simulink model "modelo_NL_DH_GUIA"  (R2025b)
settings: Solver=ode4  StartTime=0.0  StopTime=TimeXP  FixedStep=0.005  RelTol=1e-3
values from neighbouring files (symbols this model uses):
  h_ref = he    [NL_missao.m]    (also in XP_inicializacao.m = h_now; XP_missao.m = XP_msl0; XP_voo.m = XP_msl0)
  h_ref0 = h_ref    [NL_missao.m]    (also in XP_doublets_lqry2.m = 600; XP_missao.m; XP_missao_lqry.m = XP_h_ref0; XP_missao_lqry2.m = XP_h_ref0)
  h_step_final = m.h_A    [G5_sil.m]    (also in XP_voo.m = cfg(7))
  h_step_t = m.h_t(1)    [G5_sil.m]    (also in XP_voo.m = cfg(8))
  h_step_t2 = m.h_t(2)    [G5_sil.m]    (also in XP_voo.m = cfg(13))
  h_step_t3 = m.h_t(3)    [G5_sil.m]    (also in XP_voo.m = cfg(14))
  he = h_now    [XP_inicializacao.m]    (also in XP_missao.m = XP_msl0; XP_voo.m = XP_msl0)
  Kp = 0.40    (= 0.4)    [VR_replay_xp.m]    (also in XPL_probe_lat.m)
  Kq = 0.50    (= 0.5)    [VR_replay_xp.m]    (also in XPL_probe_lat.m; XP_retune_Ctheta.m = 0.1)
  psi_ref_final = deg2rad(m.psi_A)    [G5_sil.m]    (also in XP_voo.m = deg2rad(cfg(9)))
  psi_ref_t = m.psi_t(1)    [G5_sil.m]    (also in XP_voo.m = cfg(10))
  psi_ref_t2 = m.psi_t(2)    [G5_sil.m]    (also in XP_voo.m = cfg(15))
  psi_ref_t3 = m.psi_t(3)    [G5_sil.m]    (also in XP_voo.m = cfg(16))
  R_accept = cfgm.R    [NL_missao.m]    (also in XP_doublets_lqry2.m = 80; XP_missao.m = XP_R_accept; XP_missao_lqry.m = cfg_user.R; XP_missao_lqry2.m = cfg_user.R)
  theta_ref_clamp = [-0.1745  deg2rad(3)]    [XP_missao.m]    (also in XP_voo.m)
  theta_test_final = 0    [NL_missao.m]    (also in XP_missao.m = cfgm.thf)
  theta_test_init = 0    [NL_missao.m]    (also in XP_missao.m)
  theta_test_t = 1e9    (= 1000000000)    [NL_missao.m]    (also in XP_missao.m = cfgm.tht)
  TrimInput = [ctrl(4);               ctrl(1)*max_deflection;               ctrl(2)*max_deflection;               ctrl(3)*max_deflection]    [XP_inicializacao.m]    (also in XP_missao.m = [0.43; deg2rad(7.0); 0; 0]; XP_voo.m = [0.43; Ue(2); 0; 0])
  VT_ref = Ve    [NL_missao.m]    (also in XP_inicializacao.m; XP_missao.m; XP_voo.m)
  VT_ref0 = VT_ref    [NL_missao.m]    (also in XP_doublets_lqry2.m = XP_dbl_VT; XP_missao.m; XP_missao_lqry.m = 12; XP_missao_lqry2.m = 12)
  VT_step_delta = m.VT_delta    [G5_sil.m]    (also in XP_voo.m = cfg(11))
  VT_step_t = m.VT_t    [G5_sil.m]    (also in XP_voo.m = cfg(12))
  WPs = WPs_user(1,:)    [NL_missao.m]    (also in XP_doublets_lqry2.m = WPs_user; WPs(:,1:2) = ne'; XP_missao.m; XP_missao_lqry.m; XP_missao_lqry2.m)
  Xe = montaX(y)    [VR_plot_sato_real.m]    (also in VR_tic.m; plot_degrau_3vias_sato.m)
undefined symbols (not defined in the file or in its folder): act, C_alt, C_phi, C_theta, C_vel, eng, h_step_init, K_heading, Kr, psi_ref_init, tau_ref, Ve
libraries: slpidlib x4, hdlsllib x1
settings Model: Creator=anade  LastModifiedBy=kaue
settings SolverCC: ZeroCrossAlgorithm=Adaptive
settings DebuggingCC: AlgebraicLoopMsg=none  IgnoredZcDiagnostic=none

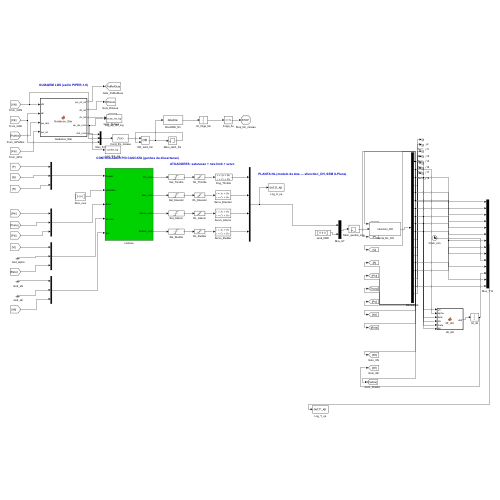
[thumbnail: Simulink's stored preview of the top-level diagram]
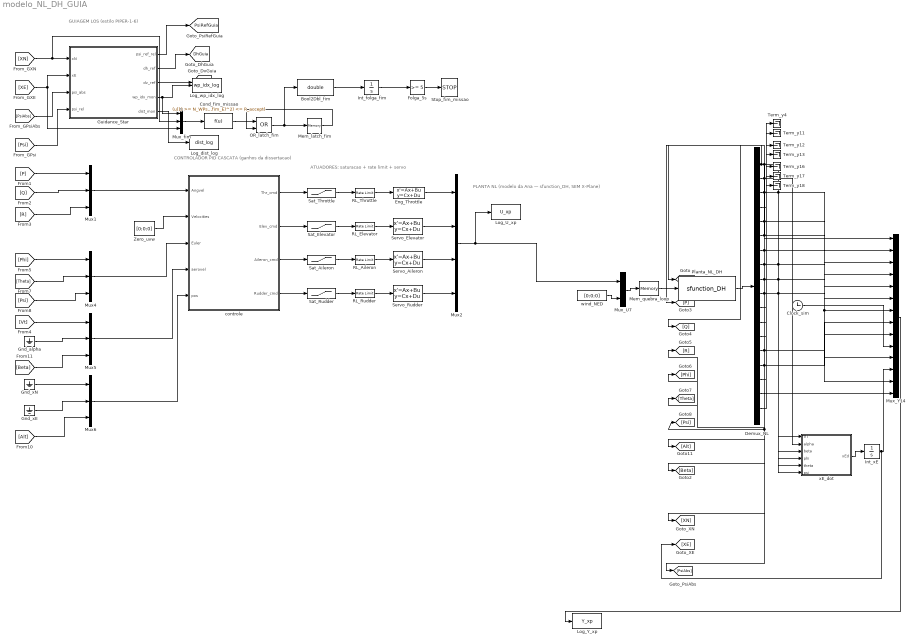
== system modelo_NL_DH_GUIA ==
  note: GUIAGEM LOS (estilo PIPER-1-6)
  note: CONTROLADOR PID CASCATA (ganhos da dissertacao)
  note: ATUADORES: saturacao + rate limit + servo
  note: PLANTA NL (modelo da Ana — sfunction_DH, SEM X-Plane)
  Bool2Dbl_fim : DataTypeConversion  OutDataTypeStr=double
  Clock_sim : Clock
  Cond_fim_missao : Fcn  Expr=(u(1) >= N_WPs) && (sqrt((u(2)-WPfim_N)^2 + (u(3)-WPfim_E)^2) <= R_accept)
  Demux_NL : Demux  Outputs=18
  Eng_Throttle : StateSpace  A=-1/eng.tau  B=1/eng.tau  D=0  InitialCondition=TrimInput(1)
  Folga_5s : hdlsllib/Logic and Bit Operations/Compare To Constant  relop=>=  const=5  OutDataTypeStr=boolean
  Gnd_alpha : Ground
  Gnd_xE : Ground
  Gnd_xN : Ground
  Guidance_Star : MATLAB Function  TreatAsAtomicUnit=on
  Int_folga_fim : Integrator
  Int_xE : Integrator
  Log_U_xp : ToWorkspace  VariableName=U_xp
  Log_Y_xp : ToWorkspace  VariableName=Y_xp
  Log_dist_log : ToWorkspace  VariableName=dist_log  SampleTime=-1
  Log_wp_idx_log : ToWorkspace  VariableName=wp_idx_log  SampleTime=-1
  Mem_latch_fim : Memory
  Mem_quebra_loop : Memory
  Mux{1,4..6} (4 alike) : Mux  Inputs=3
  Mux2 : Mux
  Mux_U7 : Mux  Inputs=2
  Mux_Y14 : Mux  Inputs=14
  Mux_fim : Mux  Inputs=3
  OR_latch_fim : Logic  Operator=OR  AllPortsSameDT=off  OutDataTypeStr=boolean
  Planta_NL_DH : S-Function  FunctionName=sfunction_DH  Parameters=Xe  SFunctionDeploymentMode=off  EnableBusSupport=off
  RL_Aileron : RateLimiter  RisingSlewLimit=act.rate  FallingSlewLimit=-act.rate  InitialCondition=TrimInput(3)
  RL_Elevator : RateLimiter  RisingSlewLimit=act.rate  FallingSlewLimit=-act.rate  InitialCondition=TrimInput(2)
  RL_Rudder : RateLimiter  RisingSlewLimit=act.rate  FallingSlewLimit=-act.rate  InitialCondition=TrimInput(4)
  RL_Throttle : RateLimiter  RisingSlewLimit=eng.rate  FallingSlewLimit=-eng.rate  InitialCondition=TrimInput(1)
  Sat_Aileron : Saturate  UpperLimit=0.4363  LowerLimit=-0.4363
  Sat_Elevator : Saturate  UpperLimit=0.4363  LowerLimit=-0.4363
  Sat_Rudder : Saturate  UpperLimit=0.4363  LowerLimit=-0.4363
  Sat_Throttle : Saturate  UpperLimit=1  LowerLimit=0
  Servo_Aileron : StateSpace  A=-act.bw  B=act.bw  D=0  InitialCondition=TrimInput(3)
  Servo_Elevator : StateSpace  A=-act.bw  B=act.bw  D=0  InitialCondition=TrimInput(2)
  Servo_Rudder : StateSpace  A=-act.bw  B=act.bw  D=0  InitialCondition=TrimInput(4)
  Stop_fim_missao : Stop
  Term_y{4,11..13,16..18} (7 alike) : Terminator
  Zero_uvw : Constant  Value=[0;0;0]
  controle : Subsystem
  wind_NED : Constant  Value=[0;0;0]
  xE_dot : MATLAB Function  TreatAsAtomicUnit=on
  tag scope: DhGuia=global, DvGuia=global, PsiRefGuia=global
  wires:
  [XN] -> Mux_fim/2, Guidance_Star/1(xN)
  [XE] -> Guidance_Star/2(xE), Mux_fim/3
  Sat_Throttle/1 -> RL_Throttle/1
  [P] -> Mux1/1
  [PsiAbs] -> Guidance_Star/3(psi_abs)
  [R] -> Mux1/3
  [Q] -> Mux1/2
  [Psi] -> Guidance_Star/4(psi_rel)
  [Phi] -> Mux4/1
  [Theta] -> Mux4/2
  [Psi] -> Mux4/3
  [Vt] -> Mux5/1
  Gnd_xN/1 -> Mux6/1
  Gnd_alpha/1 -> Mux5/2
  Mux4/1 -> controle/3(Euler)
  [Beta] -> Mux5/3
  controle/2(Elev_cmd) -> Sat_Elevator/1
  Mux5/1 -> controle/4(aerovel)
  Gnd_xE/1 -> Mux6/2
  Sat_Aileron/1 -> RL_Aileron/1
  [Alt] -> Mux6/3
  Guidance_Star/1(psi_ref_rel) -> [PsiRefGuia]
  Guidance_Star/2(dh_ref) -> [DhGuia]
  Sat_Rudder/1 -> RL_Rudder/1
  Mux1/1 -> controle/1(Angvel)
  Mux6/1 -> controle/5(pos)
  Zero_uvw/1 -> controle/2(Velocities)
  controle/1(Thr_cmd) -> Sat_Throttle/1
  controle/3(Aileron_cmd) -> Sat_Aileron/1
  controle/4(Rudder_cmd) -> Sat_Rudder/1
  Sat_Elevator/1 -> RL_Elevator/1
  Servo_Elevator/1 -> Mux2/2
  RL_Throttle/1 -> Eng_Throttle/1
  Eng_Throttle/1 -> Mux2/1
  RL_Elevator/1 -> Servo_Elevator/1
  RL_Aileron/1 -> Servo_Aileron/1
  RL_Rudder/1 -> Servo_Rudder/1
  Servo_Aileron/1 -> Mux2/3
  Servo_Rudder/1 -> Mux2/4
  Mux2/1 -> Log_U_xp/1, Mux_U7/1
  wind_NED/1 -> Mux_U7/2
  Mux_U7/1 -> Mem_quebra_loop/1
  Mem_quebra_loop/1 -> Planta_NL_DH/1
  Planta_NL_DH/1 -> Demux_NL/1
  Demux_NL/1 -> xE_dot/1(VT), Mux_Y14/1, [Vt]
  Demux_NL/3 -> xE_dot/3(beta), Mux_Y14/9, [Beta]
  Demux_NL/5 -> [P], Mux_Y14/2
  Demux_NL/6 -> [Q], Mux_Y14/3
  Demux_NL/7 -> [R], Mux_Y14/4
  Demux_NL/8 -> xE_dot/4(phi), Mux_Y14/5, [Phi]
  Demux_NL/9 -> xE_dot/5(theta), Mux_Y14/6, [Theta]
  Demux_NL/10 -> [Psi], [PsiAbs], Mux_Y14/7, Mux_Y14/13, xE_dot/6(psi)
  Demux_NL/14 -> [XN], Mux_Y14/11
  Demux_NL/15 -> [Alt], Mux_Y14/8
  Demux_NL/2 -> xE_dot/2(alpha), Mux_Y14/14
  xE_dot/1(xEd) -> Int_xE/1
  Int_xE/1 -> [XE], Mux_Y14/12
  Demux_NL/4 -> Term_y4/1
  Demux_NL/11 -> Term_y11/1
  Demux_NL/12 -> Term_y12/1
  Demux_NL/13 -> Term_y13/1
  Demux_NL/16 -> Term_y16/1
  Demux_NL/17 -> Term_y17/1
  Demux_NL/18 -> Term_y18/1
  Clock_sim/1 -> Mux_Y14/10
  Mux_Y14/1 -> Log_Y_xp/1
  Guidance_Star/3(dv_ref) -> [DvGuia]
  Guidance_Star/4(wp_idx_mon) -> Mux_fim/1, Log_wp_idx_log/1
  Guidance_Star/5(dist_mon) -> Log_dist_log/1
  Mux_fim/1 -> Cond_fim_missao/1
  Cond_fim_missao/1 -> OR_latch_fim/1
  Mem_latch_fim/1 -> OR_latch_fim/2
  OR_latch_fim/1 -> Bool2Dbl_fim/1, Mem_latch_fim/1
  Bool2Dbl_fim/1 -> Int_folga_fim/1
  Int_folga_fim/1 -> Folga_5s/1
  Folga_5s/1 -> Stop_fim_missao/1

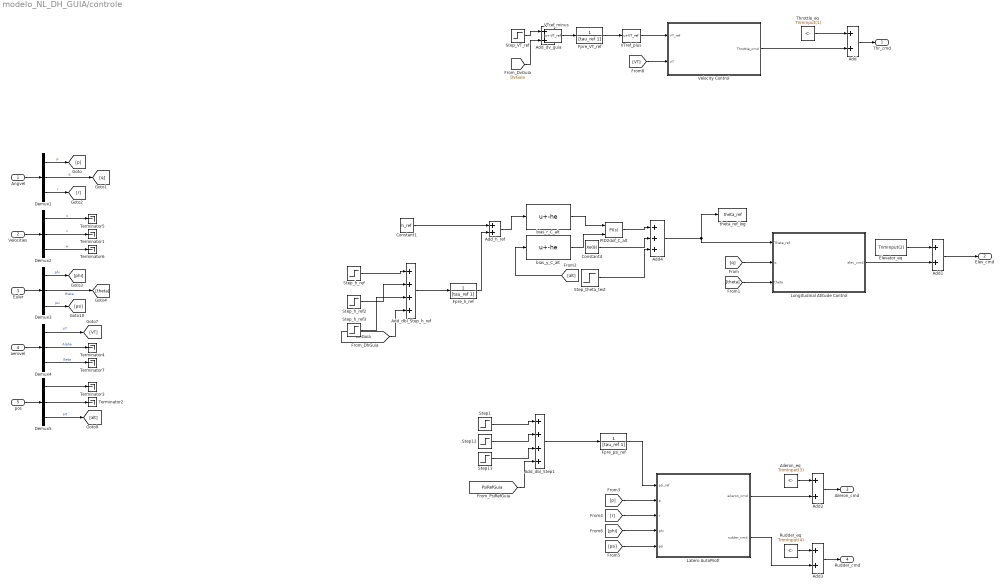
== system modelo_NL_DH_GUIA/controle ==
  Angvel : Inport
  Velocities : Inport  Port=2
  Euler : Inport  Port=3
  aerovel : Inport  Port=4
  pos : Inport  Port=5
  Add{,1..3} (4 alike) : Sum
  Add4 : Sum  Inputs=+++
  Add_dbl_Step1 : Sum  Inputs=++++
  Add_dbl_Step_h_ref : Sum  Inputs=++++
  Add_dv_guia : Sum
  Add_h_ref : Sum
  Aileron_eq : Constant  Value=TrimInput(3)
  Constant1 : Constant  Value=h_ref
  Constant4 : Constant  Value=Xe(8)
  Demux{1..5} (5 alike) : Demux  Outputs=3
  Elevator_eq : Constant  Value=TrimInput(2)
  Fpre_VT_ref : TransferFcn  Denominator=[tau_ref 1]
  Fpre_h_ref : TransferFcn  Denominator=[tau_ref 1]
  Fpre_psi_ref : TransferFcn  Denominator=[tau_ref 1]
  Latero AutoPilotl : Subsystem
  Longitudinal Atitude Control : Subsystem
  PID2dof_C_alt : slpidlib/PID Controller (2DOF)  Controller=PI  Form=Parallel  TimeDomain=Continuous-time  UseExternalTs=off  SampleTime=-1  IntegratorMethod=Forward Euler  FilterMethod=Forward Euler  ControllerParametersSource=internal  P=C_alt.Kp  I=C_alt.Ki  UseKiTs=off  D=0  UseExternalDerivativeSource=off  N=100  UseFilter=on  b=0  c=1  TunerSelectOption=Transfer Function Based (PID Tuner App)  InitialConditionSource=internal  InitialConditionForIntegrator=0  InitialConditionForFilter=0  DifferentiatorICPrevScaledInput=0  ExternalReset=none  TrackingMode=off  Kt=1  LimitOutput=on  SatLimitsSource=internal  UpperSaturationLimit=theta_ref_clamp(2)  LowerSaturationLimit=theta_ref_clamp(1)  LinearizeAsGain=on  AntiWindupMode=clamping  Kb=1  LimitIntegrator=off  UpperIntegratorSaturationLimit=inf  LowerIntegratorSaturationLimit=-inf  POutMin=[]  POutMax=[]  IOutMin=[]  IOutMax=[]  DOutMin=[]  DOutMax=[]  NOutMin=[]  NOutMax=[]  bOutMin=[]  bOutMax=[]  cOutMin=[]  cOutMax=[]  SumOutMin=[]  SumOutMax=[]  SaturationOutMin=[]  SaturationOutMax=[]  PParamMin=[]  PParamMax=[]  IParamMin=[]  IParamMax=[]  DParamMin=[]  DParamMax=[]  NParamMin=[]  NParamMax=[]  bParamMin=[]  bParamMax=[]  cParamMin=[]  cParamMax=[]  KbParamMin=[]  KbParamMax=[]  KtParamMin=[]  KtParamMax=[]  KbOutMin=[]  KbOutMax=[]  KtOutMin=[]  KtOutMax=[]  IntegratorOutMin=[]  IntegratorOutMax=[]  FilterOutMin=[]  FilterOutMax=[]  SumI1OutMin=[]  SumI1OutMax=[]  SumI2OutMin=[]  SumI2OutMax=[]  SumI3OutMin=[]  SumI3OutMax=[]  SumI4OutMin=[]  SumI4OutMax=[]  SumDOutMin=[]  SumDOutMax=[]  Sum1OutMin=[]  Sum1OutMax=[]  Sum2OutMin=[]  Sum2OutMax=[]  Sum3OutMin=[]  Sum3OutMax=[]  DifferentiatorOutMin=[]  DifferentiatorOutMax=[]  FilterDiffOutCoefMin=[]  FilterDiffOutCoefMax=[]  ReciprocalOutMin=[]  ReciprocalOutMax=[]  SumDenOutMin=[]  SumDenOutMax=[]  SumNumOutMin=[]  SumNumOutMax=[]  DivideOutMin=[]  DivideOutMax=[]  UdiffTsProdOutMin=[]  UdiffTsProdOutMax=[]  NTsProdOutMin=[]  NTsProdOutMax=[]  UintegralTsProdOutMin=[]  UintegralTsProdOutMax=[]  UngainTsProdOutMin=[]  UngainTsProdOutMax=[]  ClampingZeroOutDataTypeStr=Inherit: Inherit via back propagation  ClampingZeroOutMin=[]  ClampingZeroOutMax=[]  FilterDenConstantOutDataTypeStr=Inherit: Inherit via back propagation  FilterDenConstantOutMin=[]  FilterDenConstantOutMax=[]  PCopyOutDataTypeStr=Inherit: Inherit via back propagation  PCopyOutMin=[]  PCopyOutMax=[]  NCopyOutDataTypeStr=Inherit: Inherit via back propagation  NCopyOutMin=[]  NCopyOutMax=[]  IntegratorContinuousStateAttributes=''  IntegratorStateMustResolveToSignalObject=off  IntegratorRTWStateStorageClass=Auto  FilterContinuousStateAttributes=''  FilterStateMustResolveToSignalObject=off  FilterRTWStateStorageClass=Auto  ParallelPVariant=InternalParameters  IdealPVariant=Disabled  IVariant=InternalParameters  DVariant=Disabled  bVariant=InternalParameters  cVariant=Disabled  IntegratorVariant=Continuous  SatVariant=Enabled  AWVariant=ContClampingParallel  PCopyVariant=Disabled  TRVariant=Disabled  FdbkBlocksVariant=Forward  IdealPFdbkVariant=Disabled  SatFdbkVariant=Disabled  DerivativeFilterVariant=Disabled  NVariant=Disabled  NCopyVariant=Disabled_SignalSpec  FilterICVariant=Disabled  IntegratorICVariant=InternalICs  ExternalResetVariant=Disabled  TRSumVariant=Passthrough  SumFdbkVariant=Disabled  SumVariant=Sum_PI  TsampFilterVariant=InternalTs  TsampNgainVariant=Passthrough  TsampIntegralVariant=Disabled_SignalSpec  ExternalSaturationOutDataTypeStr=Inherit: Same as second input  DerivativeSourceVariant=Disabled  PreIntVariant=InternalPreInt
  Rudder_eq : Constant  Value=TrimInput(4)
  Step1 : Step  Time=psi_ref_t  Before=psi_ref_init  After=psi_ref_final  SampleTime=0
  Step12 : Step  Time=psi_ref_t2  After=-2*psi_ref_final  SampleTime=0
  Step13 : Step  Time=psi_ref_t3  After=psi_ref_final  SampleTime=0
  Step_VT_ref : Step  Time=VT_step_t  Before=VT_ref  After=VT_ref+VT_step_delta  SampleTime=0
  Step_h_ref : Step  Time=h_step_t  Before=h_step_init  After=h_step_final  SampleTime=0
  Step_h_ref2 : Step  Time=h_step_t2  After=-2*h_step_final  SampleTime=0
  Step_h_ref3 : Step  Time=h_step_t3  After=h_step_final  SampleTime=0
  Step_theta_test : Step  Time=theta_test_t  Before=theta_test_init  After=theta_test_final  SampleTime=0
  Terminator{1..7} (7 alike) : Terminator
  Throttle_eq : Constant  Value=TrimInput(1)
  VTref_minus : Bias  Bias=-VT_ref
  VTref_plus : Bias  Bias=VT_ref
  Velocity Control : Subsystem
  bias_r_C_alt : Bias  Bias=-he  SaturateOnIntegerOverflow=off
  bias_y_C_alt : Bias  Bias=-he  SaturateOnIntegerOverflow=off
  theta_ref_log : ToWorkspace  VariableName=theta_ref  SaveFormat=Structure With Time  SampleTime=-1
  Thr_cmd : Outport
  Elev_cmd : Outport  Port=2
  Aileron_cmd : Outport  Port=3
  Rudder_cmd : Outport  Port=4
  wires:
  Angvel/1 -> Demux1/1
  Velocities/1 -> Demux2/1
  Demux1/1 -> [p]  "p"
  Demux1/2 -> [q]  "q"
  Demux1/3 -> [r]  "r"
  Euler/1 -> Demux3/1
  Demux3/3 -> [psi]  "psi"
  Demux3/1 -> [phi]  "phi"
  Demux3/2 -> [theta]  "theta"
  Demux2/3 -> Terminator6/1  "w"
  Demux2/1 -> Terminator5/1  "u"
  Demux2/2 -> Terminator1/1  "v"
  [theta] -> Longitudinal Atitude Control/3(theta)
  aerovel/1 -> Demux4/1
  Demux4/1 -> [VT]  "VT"
  Demux4/2 -> Terminator4/1  "Alpha"
  Demux4/3 -> Terminator7/1  "Beta"
  [q] -> Longitudinal Atitude Control/2(q)
  [VT] -> Velocity Control/2(VT)
  pos/1 -> Demux5/1
  Demux5/3 -> [alt]  "alt"
  Demux5/2 -> Terminator2/1
  Demux5/1 -> Terminator3/1
  [p] -> Latero AutoPilotl/2(p)
  [r] -> Latero AutoPilotl/3(r)
  [psi] -> Latero AutoPilotl/5(psi)
  [phi] -> Latero AutoPilotl/4(phi)
  Constant4/1 -> Add4/2
  Add1/1 -> Elev_cmd/1
  Longitudinal Atitude Control/1(elev_cmd) -> Add1/2
  Add/1 -> Thr_cmd/1
  Velocity Control/1(Throttle_cmd) -> Add/2
  Latero AutoPilotl/1(aileron_cmd) -> Add2/2
  Elevator_eq/1 -> Add1/1
  Rudder_eq/1 -> Add3/1
  Aileron_eq/1 -> Add2/1
  Latero AutoPilotl/2(rudder_cmd) -> Add3/2
  Add2/1 -> Aileron_cmd/1
  Add3/1 -> Rudder_cmd/1
  Throttle_eq/1 -> Add/1
  Add4/1 -> theta_ref_log/1, Longitudinal Atitude Control/1(Theta_ref)
  Constant1/1 -> Add_h_ref/1
  Step_h_ref/1 -> Add_dbl_Step_h_ref/1
  Step_h_ref2/1 -> Add_dbl_Step_h_ref/2
  Step_h_ref3/1 -> Add_dbl_Step_h_ref/3
  Step1/1 -> Add_dbl_Step1/1
  Step12/1 -> Add_dbl_Step1/2
  Step13/1 -> Add_dbl_Step1/3
  Add_dbl_Step_h_ref/1 -> Fpre_h_ref/1
  Fpre_h_ref/1 -> Add_h_ref/2
  Add_dbl_Step1/1 -> Fpre_psi_ref/1
  Fpre_psi_ref/1 -> Latero AutoPilotl/1(psi_ref)
  VTref_minus/1 -> Fpre_VT_ref/1
  Fpre_VT_ref/1 -> VTref_plus/1
  VTref_plus/1 -> Velocity Control/1(VT_ref)
  Add_h_ref/1 -> bias_r_C_alt/1
  [alt] -> bias_y_C_alt/1
  bias_r_C_alt/1 -> PID2dof_C_alt/1
  bias_y_C_alt/1 -> PID2dof_C_alt/2
  PID2dof_C_alt/1 -> Add4/1
  [PsiRefGuia] -> Add_dbl_Step1/4
  [DhGuia] -> Add_dbl_Step_h_ref/4
  Step_VT_ref/1 -> Add_dv_guia/1
  [DvGuia] -> Add_dv_guia/2
  Add_dv_guia/1 -> VTref_minus/1
  Step_theta_test/1 -> Add4/3

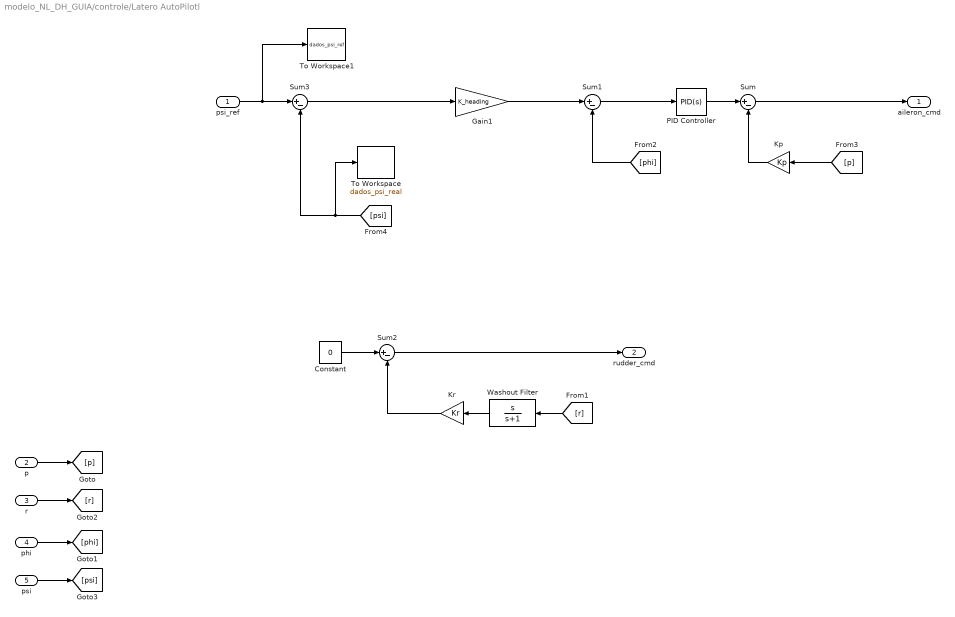
== system modelo_NL_DH_GUIA/controle/Latero AutoPilotl ==
  psi_ref : Inport
  p : Inport  Port=2
  r : Inport  Port=3
  phi : Inport  Port=4
  psi : Inport  Port=5
  Constant : Constant  Value=0
  Gain1 : Gain  Gain=K_heading
  Kp : Gain  Gain=Kp
  Kr : Gain  Gain=Kr
  PID Controller : slpidlib/PID Controller  Controller=PID  Form=Parallel  TimeDomain=Continuous-time  UseExternalTs=off  SampleTime=-1  IntegratorMethod=Forward Euler  FilterMethod=Forward Euler  ControllerParametersSource=internal  P=C_phi.Kp  I=C_phi.Ki  UseKiTs=off  D=C_phi.Kd  UseExternalDerivativeSource=off  N=C_phi.N  UseFilter=on  TunerSelectOption=Transfer Function Based (PID Tuner App)  InitialConditionSource=internal  InitialConditionForIntegrator=0  InitialConditionForFilter=0  DifferentiatorICPrevScaledInput=0  ExternalReset=none  TrackingMode=off  Kt=1  LimitOutput=on  SatLimitsSource=internal  UpperSaturationLimit=0.4363  LowerSaturationLimit=-0.4363  LinearizeAsGain=on  AntiWindupMode=clamping  Kb=1  LimitIntegrator=off  UpperIntegratorSaturationLimit=inf  LowerIntegratorSaturationLimit=-inf  POutMin=[]  POutMax=[]  IOutMin=[]  IOutMax=[]  DOutMin=[]  DOutMax=[]  NOutMin=[]  NOutMax=[]  SumOutMin=[]  SumOutMax=[]  SaturationOutMin=[]  SaturationOutMax=[]  PParamMin=[]  PParamMax=[]  IParamMin=[]  IParamMax=[]  DParamMin=[]  DParamMax=[]  NParamMin=[]  NParamMax=[]  KbParamMin=[]  KbParamMax=[]  KtParamMin=[]  KtParamMax=[]  KbOutMin=[]  KbOutMax=[]  KtOutMin=[]  KtOutMax=[]  IntegratorOutMin=[]  IntegratorOutMax=[]  FilterOutMin=[]  FilterOutMax=[]  SumI1OutMin=[]  SumI1OutMax=[]  SumI2OutMin=[]  SumI2OutMax=[]  SumI3OutMin=[]  SumI3OutMax=[]  SumI4OutMin=[]  SumI4OutMax=[]  SumDOutMin=[]  SumDOutMax=[]  DifferentiatorOutMin=[]  DifferentiatorOutMax=[]  FilterDiffOutCoefMin=[]  FilterDiffOutCoefMax=[]  ReciprocalOutMin=[]  ReciprocalOutMax=[]  SumDenOutMin=[]  SumDenOutMax=[]  SumNumOutMin=[]  SumNumOutMax=[]  DivideOutMin=[]  DivideOutMax=[]  UdiffTsProdOutMin=[]  UdiffTsProdOutMax=[]  NTsProdOutMin=[]  NTsProdOutMax=[]  UintegralTsProdOutMin=[]  UintegralTsProdOutMax=[]  UngainTsProdOutMin=[]  UngainTsProdOutMax=[]  ClampingZeroOutDataTypeStr=Inherit: Inherit via back propagation  ClampingZeroOutMin=[]  ClampingZeroOutMax=[]  FilterDenConstantOutDataTypeStr=Inherit: Inherit via back propagation  FilterDenConstantOutMin=[]  FilterDenConstantOutMax=[]  PCopyOutDataTypeStr=Inherit: Inherit via back propagation  PCopyOutMin=[]  PCopyOutMax=[]  NCopyOutDataTypeStr=Inherit: Inherit via back propagation  NCopyOutMin=[]  NCopyOutMax=[]  IntegratorContinuousStateAttributes=''  IntegratorStateMustResolveToSignalObject=off  IntegratorRTWStateStorageClass=Auto  FilterContinuousStateAttributes=''  FilterStateMustResolveToSignalObject=off  FilterRTWStateStorageClass=Auto  ParallelPVariant=InternalParameters  IdealPVariant=Disabled  IVariant=InternalParameters  DVariant=InternalParameters  IntegratorVariant=Continuous  SatVariant=Enabled  AWVariant=ContClampingParallel  PCopyVariant=Disabled  TRVariant=Disabled  FdbkBlocksVariant=Forward  IdealPFdbkVariant=Disabled  SatFdbkVariant=Disabled  DerivativeFilterVariant=ContFilter  NVariant=InternalParameters  NCopyVariant=Disabled  FilterICVariant=InternalICsFilter  IntegratorICVariant=InternalICs  ExternalResetVariant=Disabled  TRSumVariant=Passthrough  SumFdbkVariant=Disabled  SumVariant=Sum_PID  TsampFilterVariant=InternalTs  TsampNgainVariant=Passthrough  TsampIntegralVariant=Disabled_SignalSpec  ExternalSaturationOutDataTypeStr=Inherit: Same as second input  DerivativeSourceVariant=ErrorSignal  PreIntVariant=InternalPreInt
  Sum{,1..3} (4 alike) : Sum  Inputs=|+-
  To Workspace : ToWorkspace  VariableName=dados_psi_real  SaveFormat=Timeseries  SampleTime=-1
      settings: Save2DSignal=2-D array (concatenate along first dimension)
  To Workspace1 : ToWorkspace  VariableName=dados_psi_ref  SaveFormat=Timeseries  SampleTime=-1
      settings: Save2DSignal=2-D array (concatenate along first dimension)
  Washout Filter : TransferFcn  Numerator=[1 0]  Denominator=[1 1]
  aileron_cmd : Outport
  rudder_cmd : Outport  Port=2
  wires:
  [p] -> Kp/1
  [phi] -> Sum1/2
  Kp/1 -> Sum/2
  PID Controller/1 -> Sum/1
  p/1 -> [p]
  [r] -> Washout Filter/1
  Kr/1 -> Sum2/2
  r/1 -> [r]
  Washout Filter/1 -> Kr/1
  phi/1 -> [phi]
  psi/1 -> [psi]
  Sum3/1 -> Gain1/1
  [psi] -> Sum3/2, To Workspace/1
  psi_ref/1 -> Sum3/1, To Workspace1/1
  Sum2/1 -> rudder_cmd/1
  Constant/1 -> Sum2/1
  Gain1/1 -> Sum1/1
  Sum/1 -> aileron_cmd/1
  Sum1/1 -> PID Controller/1

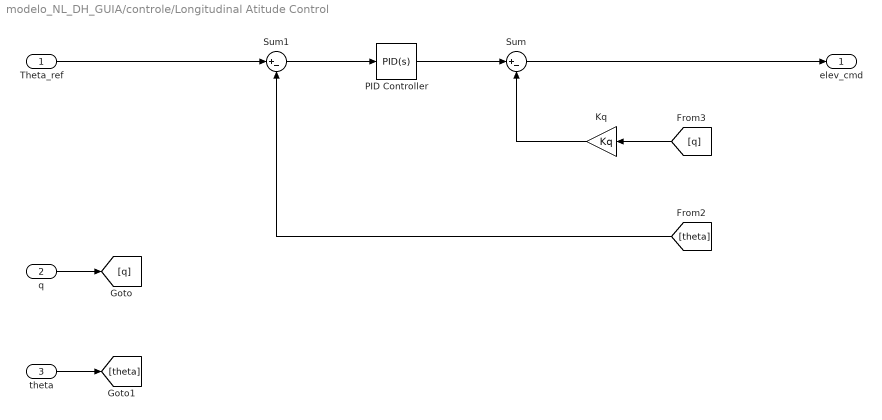
== system modelo_NL_DH_GUIA/controle/Longitudinal Atitude Control ==
  Theta_ref : Inport
  q : Inport  Port=2
  theta : Inport  Port=3
  Kq : Gain  Gain=Kq
  PID Controller : slpidlib/PID Controller  Controller=PID  Form=Parallel  TimeDomain=Continuous-time  UseExternalTs=off  SampleTime=-1  IntegratorMethod=Forward Euler  FilterMethod=Forward Euler  ControllerParametersSource=internal  P=C_theta.Kp  I=C_theta.Ki  UseKiTs=off  D=C_theta.Kd  UseExternalDerivativeSource=off  N=C_theta.N  UseFilter=on  TunerSelectOption=Transfer Function Based (PID Tuner App)  InitialConditionSource=internal  InitialConditionForIntegrator=0  InitialConditionForFilter=0  DifferentiatorICPrevScaledInput=0  ExternalReset=none  TrackingMode=off  Kt=1  LimitOutput=on  SatLimitsSource=internal  UpperSaturationLimit=0.4363  LowerSaturationLimit=-0.4363  LinearizeAsGain=on  AntiWindupMode=clamping  Kb=1  LimitIntegrator=off  UpperIntegratorSaturationLimit=inf  LowerIntegratorSaturationLimit=-inf  POutMin=[]  POutMax=[]  IOutMin=[]  IOutMax=[]  DOutMin=[]  DOutMax=[]  NOutMin=[]  NOutMax=[]  SumOutMin=[]  SumOutMax=[]  SaturationOutMin=[]  SaturationOutMax=[]  PParamMin=[]  PParamMax=[]  IParamMin=[]  IParamMax=[]  DParamMin=[]  DParamMax=[]  NParamMin=[]  NParamMax=[]  KbParamMin=[]  KbParamMax=[]  KtParamMin=[]  KtParamMax=[]  KbOutMin=[]  KbOutMax=[]  KtOutMin=[]  KtOutMax=[]  IntegratorOutMin=[]  IntegratorOutMax=[]  FilterOutMin=[]  FilterOutMax=[]  SumI1OutMin=[]  SumI1OutMax=[]  SumI2OutMin=[]  SumI2OutMax=[]  SumI3OutMin=[]  SumI3OutMax=[]  SumI4OutMin=[]  SumI4OutMax=[]  SumDOutMin=[]  SumDOutMax=[]  DifferentiatorOutMin=[]  DifferentiatorOutMax=[]  FilterDiffOutCoefMin=[]  FilterDiffOutCoefMax=[]  ReciprocalOutMin=[]  ReciprocalOutMax=[]  SumDenOutMin=[]  SumDenOutMax=[]  SumNumOutMin=[]  SumNumOutMax=[]  DivideOutMin=[]  DivideOutMax=[]  UdiffTsProdOutMin=[]  UdiffTsProdOutMax=[]  NTsProdOutMin=[]  NTsProdOutMax=[]  UintegralTsProdOutMin=[]  UintegralTsProdOutMax=[]  UngainTsProdOutMin=[]  UngainTsProdOutMax=[]  ClampingZeroOutDataTypeStr=Inherit: Inherit via back propagation  ClampingZeroOutMin=[]  ClampingZeroOutMax=[]  FilterDenConstantOutDataTypeStr=Inherit: Inherit via back propagation  FilterDenConstantOutMin=[]  FilterDenConstantOutMax=[]  PCopyOutDataTypeStr=Inherit: Inherit via back propagation  PCopyOutMin=[]  PCopyOutMax=[]  NCopyOutDataTypeStr=Inherit: Inherit via back propagation  NCopyOutMin=[]  NCopyOutMax=[]  IntegratorContinuousStateAttributes=''  IntegratorStateMustResolveToSignalObject=off  IntegratorRTWStateStorageClass=Auto  FilterContinuousStateAttributes=''  FilterStateMustResolveToSignalObject=off  FilterRTWStateStorageClass=Auto  ParallelPVariant=InternalParameters  IdealPVariant=Disabled  IVariant=InternalParameters  DVariant=InternalParameters  IntegratorVariant=Continuous  SatVariant=Enabled  AWVariant=ContClampingParallel  PCopyVariant=Disabled  TRVariant=Disabled  FdbkBlocksVariant=Forward  IdealPFdbkVariant=Disabled  SatFdbkVariant=Disabled  DerivativeFilterVariant=ContFilter  NVariant=InternalParameters  NCopyVariant=Disabled  FilterICVariant=InternalICsFilter  IntegratorICVariant=InternalICs  ExternalResetVariant=Disabled  TRSumVariant=Passthrough  SumFdbkVariant=Disabled  SumVariant=Sum_PID  TsampFilterVariant=InternalTs  TsampNgainVariant=Passthrough  TsampIntegralVariant=Disabled_SignalSpec  ExternalSaturationOutDataTypeStr=Inherit: Same as second input  DerivativeSourceVariant=ErrorSignal  PreIntVariant=InternalPreInt
  Sum : Sum  Inputs=|+-
  Sum1 : Sum  Inputs=|+-
  elev_cmd : Outport
  wires:
  Sum1/1 -> PID Controller/1
  Sum/1 -> elev_cmd/1
  [q] -> Kq/1
  [theta] -> Sum1/2
  Kq/1 -> Sum/2
  PID Controller/1 -> Sum/1
  theta/1 -> [theta]
  q/1 -> [q]
  Theta_ref/1 -> Sum1/1

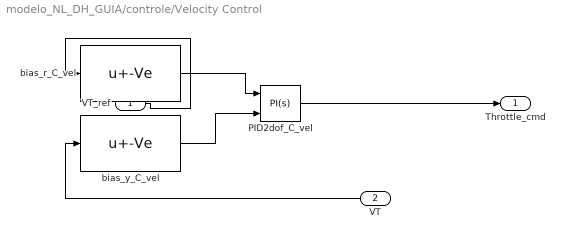
== system modelo_NL_DH_GUIA/controle/Velocity Control ==
  VT_ref : Inport
  VT : Inport  Port=2
  PID2dof_C_vel : slpidlib/PID Controller (2DOF)  Controller=PI  Form=Parallel  TimeDomain=Continuous-time  UseExternalTs=off  SampleTime=-1  IntegratorMethod=Forward Euler  FilterMethod=Forward Euler  ControllerParametersSource=internal  P=C_vel.Kp  I=C_vel.Ki  UseKiTs=off  D=0  UseExternalDerivativeSource=off  N=100  UseFilter=on  b=0  c=1  TunerSelectOption=Transfer Function Based (PID Tuner App)  InitialConditionSource=internal  InitialConditionForIntegrator=0  InitialConditionForFilter=0  DifferentiatorICPrevScaledInput=0  ExternalReset=none  TrackingMode=off  Kt=1  LimitOutput=on  SatLimitsSource=internal  UpperSaturationLimit=0.51  LowerSaturationLimit=-0.49  LinearizeAsGain=on  AntiWindupMode=clamping  Kb=1  LimitIntegrator=off  UpperIntegratorSaturationLimit=inf  LowerIntegratorSaturationLimit=-inf  POutMin=[]  POutMax=[]  IOutMin=[]  IOutMax=[]  DOutMin=[]  DOutMax=[]  NOutMin=[]  NOutMax=[]  bOutMin=[]  bOutMax=[]  cOutMin=[]  cOutMax=[]  SumOutMin=[]  SumOutMax=[]  SaturationOutMin=[]  SaturationOutMax=[]  PParamMin=[]  PParamMax=[]  IParamMin=[]  IParamMax=[]  DParamMin=[]  DParamMax=[]  NParamMin=[]  NParamMax=[]  bParamMin=[]  bParamMax=[]  cParamMin=[]  cParamMax=[]  KbParamMin=[]  KbParamMax=[]  KtParamMin=[]  KtParamMax=[]  KbOutMin=[]  KbOutMax=[]  KtOutMin=[]  KtOutMax=[]  IntegratorOutMin=[]  IntegratorOutMax=[]  FilterOutMin=[]  FilterOutMax=[]  SumI1OutMin=[]  SumI1OutMax=[]  SumI2OutMin=[]  SumI2OutMax=[]  SumI3OutMin=[]  SumI3OutMax=[]  SumI4OutMin=[]  SumI4OutMax=[]  SumDOutMin=[]  SumDOutMax=[]  Sum1OutMin=[]  Sum1OutMax=[]  Sum2OutMin=[]  Sum2OutMax=[]  Sum3OutMin=[]  Sum3OutMax=[]  DifferentiatorOutMin=[]  DifferentiatorOutMax=[]  FilterDiffOutCoefMin=[]  FilterDiffOutCoefMax=[]  ReciprocalOutMin=[]  ReciprocalOutMax=[]  SumDenOutMin=[]  SumDenOutMax=[]  SumNumOutMin=[]  SumNumOutMax=[]  DivideOutMin=[]  DivideOutMax=[]  UdiffTsProdOutMin=[]  UdiffTsProdOutMax=[]  NTsProdOutMin=[]  NTsProdOutMax=[]  UintegralTsProdOutMin=[]  UintegralTsProdOutMax=[]  UngainTsProdOutMin=[]  UngainTsProdOutMax=[]  ClampingZeroOutDataTypeStr=Inherit: Inherit via back propagation  ClampingZeroOutMin=[]  ClampingZeroOutMax=[]  FilterDenConstantOutDataTypeStr=Inherit: Inherit via back propagation  FilterDenConstantOutMin=[]  FilterDenConstantOutMax=[]  PCopyOutDataTypeStr=Inherit: Inherit via back propagation  PCopyOutMin=[]  PCopyOutMax=[]  NCopyOutDataTypeStr=Inherit: Inherit via back propagation  NCopyOutMin=[]  NCopyOutMax=[]  IntegratorContinuousStateAttributes=''  IntegratorStateMustResolveToSignalObject=off  IntegratorRTWStateStorageClass=Auto  FilterContinuousStateAttributes=''  FilterStateMustResolveToSignalObject=off  FilterRTWStateStorageClass=Auto  ParallelPVariant=InternalParameters  IdealPVariant=Disabled  IVariant=InternalParameters  DVariant=Disabled  bVariant=InternalParameters  cVariant=Disabled  IntegratorVariant=Continuous  SatVariant=Enabled  AWVariant=ContClampingParallel  PCopyVariant=Disabled  TRVariant=Disabled  FdbkBlocksVariant=Forward  IdealPFdbkVariant=Disabled  SatFdbkVariant=Disabled  DerivativeFilterVariant=Disabled  NVariant=Disabled  NCopyVariant=Disabled_SignalSpec  FilterICVariant=Disabled  IntegratorICVariant=InternalICs  ExternalResetVariant=Disabled  TRSumVariant=Passthrough  SumFdbkVariant=Disabled  SumVariant=Sum_PI  TsampFilterVariant=InternalTs  TsampNgainVariant=Passthrough  TsampIntegralVariant=Disabled_SignalSpec  ExternalSaturationOutDataTypeStr=Inherit: Same as second input  DerivativeSourceVariant=Disabled  PreIntVariant=InternalPreInt
  bias_r_C_vel : Bias  Bias=-Ve  SaturateOnIntegerOverflow=off
  bias_y_C_vel : Bias  Bias=-Ve  SaturateOnIntegerOverflow=off
  Throttle_cmd : Outport
  wires:
  VT_ref/1 -> bias_r_C_vel/1
  VT/1 -> bias_y_C_vel/1
  bias_r_C_vel/1 -> PID2dof_C_vel/1
  bias_y_C_vel/1 -> PID2dof_C_vel/2
  PID2dof_C_vel/1 -> Throttle_cmd/1

== matlab function modelo_NL_DH_GUIA/xE_dot ==
  data: VT input; xEd output; alpha input; beta input; phi input; theta input; psi input
function xEd = xE_dot(VT, alpha, beta, phi, theta, psi)
% velocidade Leste inercial reconstruida das saidas do observador
% (exato p/ vento zero): [u v w] do triedro aerodinamico -> Lnb linha 2.
u = VT*cos(alpha)*cos(beta); v = VT*sin(beta); w = VT*sin(alpha)*cos(beta);
xEd = (sin(phi)*sin(theta)*sin(psi)+cos(phi)*cos(psi))*v ...
    + (cos(phi)*sin(theta)*sin(psi)-sin(phi)*cos(psi))*w ...
    + cos(theta)*sin(psi)*u;
end

== matlab function modelo_NL_DH_GUIA/Guidance_Star ==
  settings: updateMethod=DISCRETE  sampleTime=0.05
  data: xN input; psi_ref_rel output; xE input; psi_abs input; psi_rel input; dh_ref output; dv_ref output; wp_idx_mon output; dist_mon output; WPs parameter; R_accept parameter; h_ref0 parameter; VT_ref0 parameter
function [psi_ref_rel, dh_ref, dv_ref, wp_idx_mon, dist_mon] = Guidance_Star(xN, xE, psi_abs, psi_rel, WPs, R_accept, h_ref0, VT_ref0)
% Guiagem por waypoints LOS — portado de chart_44 (Guidance_Star) do
% NL_guidance do Julio Machado (PIPER-1-6), adaptado ao harness do DH:
%   - WPs = [Norte(m) Leste(m) Alt MSL(m) Vel(m/s)]; posicao NE relativa
%     ao ENGATE (canais 11-12 do xp_read_dh), LOS em NE absoluto;
%   - wp_idx inicia em 1 (nosso WP1 ja e' o primeiro ALVO; o Julio
%     nascia sobre o WP1 e mirava o 2);
%   - troca de WP: dist <= R_accept && wp_idx < num_wps (segura o ultimo);
%   - psi_los e' proa ABSOLUTA; o harness trabalha com proa RELATIVA ao
%     engate (unwrap continuo, canal 7). Conversao SEM tocar no controle:
%       psi_ref_rel = psi_rel + wrap(psi_los - psi_abs)
%     com wrap(x)=mod(x+pi,2pi)-pi (o calc_erro_proa do Julio) — o erro
%     que chega ao heading hold e' o mesmo, na convencao relativa.
%   - saidas dh_ref/dv_ref sao DELTAS sobre h_ref0/VT_ref0 (as refs de
%     engate do workspace): entram nos pontos dos doublets ja existentes
%     e passam pelos pre-filtros tau_ref do modelo (suavizacao de troca).
persistent wp_idx hold_psi
if isempty(wp_idx), wp_idx = 1; hold_psi = NaN; end
num_wps = size(WPs, 1);
if wp_idx > num_wps, wp_idx = num_wps; end
dist = sqrt((WPs(wp_idx,1) - xN)^2 + (WPs(wp_idx,2) - xE)^2);
if (dist <= R_accept)
    if wp_idx < num_wps
        wp_idx = wp_idx + 1;
    elseif isnan(hold_psi)
        % ADAPTACAO ao DH (difere do Julio, que orbita o ultimo
        % WP): orbitar com LOS puro vira curva continua apertada
        % e o DH nao tem margem de energia p/ isso (G1 2026-08-20:
        % phi 30-50, VT<9). Apos capturar o ULTIMO WP, congela a
        % proa da captura — voo reto nivelado ate o tempo esgotar.
        hold_psi = psi_rel;
    end
end
tN = WPs(wp_idx, 1);
tE = WPs(wp_idx, 2);
psi_los = atan2(tE - xE, tN - xN);
dpsi = mod(psi_los - psi_abs + pi, 2*pi) - pi;
if isnan(hold_psi)
    psi_ref_rel = psi_rel + dpsi;
else
    psi_ref_rel = hold_psi;
end
dh_ref = WPs(wp_idx, 3) - h_ref0;
dv_ref = WPs(wp_idx, 4) - VT_ref0;
wp_idx_mon = wp_idx;
dist_mon = dist;
end
